simulink model "sampleModel1883"  (R2023a)
settings: Solver=VariableStepAuto  StartTime=0.0  StopTime=10.0  RelTol=1e-3
libraries: hdlsllib x1
settings Model: Creator=user1  LastModifiedBy=user1

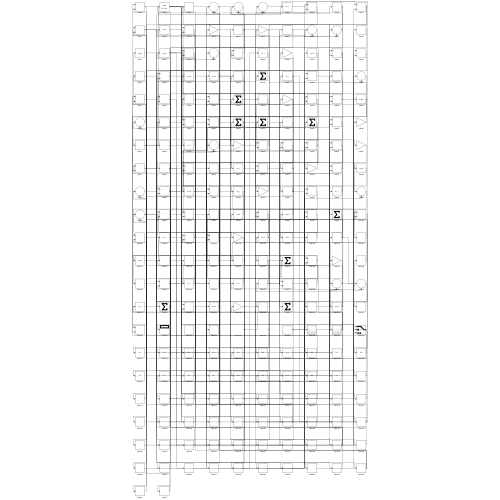
[thumbnail: Simulink's stored preview of the top-level diagram]
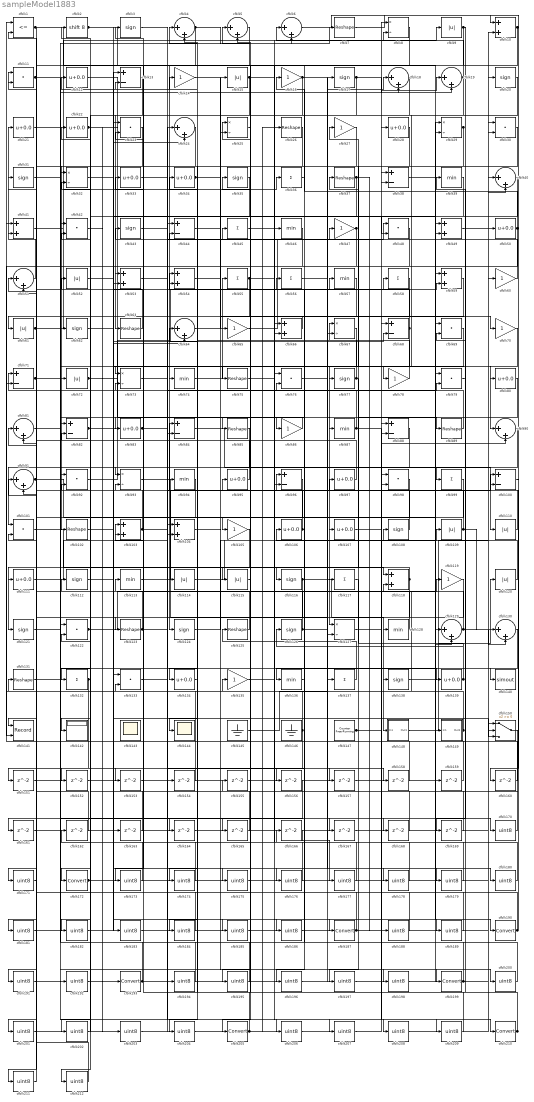
== system sampleModel1883 ==
  cfblk1 : RelationalOperator  Operator=<=  OutDataTypeStr=boolean  InputSameDT=off
  cfblk{10,41,49,53..54,59,66,103..104,118} (10 alike) : Sum
  cfblk{13,38,44,68,71,82,84,88,96,100} (10 alike) : Sum  Inputs=+-
  cfblk{11,23,30,42,48,69,76,79,92,98,101,122,133} (13 alike) : DotProduct  OutDataTypeStr=Inherit: Inherit via internal rule
  cfblk{7,26,37,63,75,85,89,102,123,125,131} (11 alike) : Reshape
  cfblk{14,16,27,47,60,65,70,78,86,105,119,135} (12 alike) : Gain
  cfblk{12,21..22,28,33..34,50,80,83,95,97,106..107,111,134,139} (16 alike) : Bias  Bias=0.0  SaturateOnIntegerOverflow=off
  cfblk{3,17,20,31,35,43,62,77,108,112,116,121,124,126,138} (15 alike) : Signum
  cfblk{9,15,52,61,72,109..110,114..115,120} (10 alike) : Abs  SaturateOnIntegerOverflow=off
  cfblk{39,46,57,74,87,94,113,128,136} (9 alike) : MinMax
  cfblk{36,45,55..56,58,99,117,132,137} (9 alike) : Sum  Inputs=+
  cfblk{8,25,29,32,67,73,93,127} (8 alike) : Product  Inputs=*/  RndMeth=Zero  SaturateOnIntegerOverflow=on
  cfblk{4..6,18..19,24,40,51,64,81,90..91,129..130} (14 alike) : Sum  Inputs=|++
  cfblk140 : ToWorkspace  VariableName=simout  SaveFormat=Timeseries  SampleTime=-1
  cfblk141 : Record  FileSettingsInternal="{\"entries\":[{\"content\":{\"excelSettings\":{\"content\":{},\"type\":\"Streamout.ExcelSettings\"}},\"type\":\"Streamout.FileSettingStorage\",\"uuid\":\"\"}],\"packageUris\":[\"http:\\/\\/schema.mathworks.com\\/mf0\\/streamout_blocks\\/R2020a\"],\"version\":\"1.0\"}"  Layout=[1 1]  SignalsInternal="{\"entries\":[{\"content\":{\"signals\":[{\"content\":{\"blockPath\":[],\"dimensions\":[1],\"domain\":\"\",\"lineColor\":\"#a2142f\",\"plots\":[1],\"port\":1,\"signalID\":4777,\"signalName\":\"XY Graph:1\"},\"type\":\"RecordBlkView.Signal\",\"uuid\":\"\"},{\"content\":{\"blockPath\":[],\"dimensions\":[1],\"domain\":\"\",\"lineColor\":\"#139fff\",\"plots\":[1],\"port\":2,\"signalID\":4780,\"signalName\":\"XY Graph:2\"},\"type\":\"RecordBlkView.Signal\",\"uuid\":\"\"}]},\"type\":\"RecordBlkView.InputSignals\",\"uuid\":\"\"}],\"packageUris\":[\"http:\\/\\/schema.mathworks.com\\/mf0\\/streamout_blocks\\/R2020a\"],\"version\":\"1.0\"}"  VisualizationBindings="{\"xyplotplugin\":{\"info\":[{\"series\":[{\"bindingParametersList\":[{\"parameter\":\"X-Axis\",\"signalID\":4777,\"signalName\":\"XY Graph:1\"},{\"parameter\":\"Y-Axis\",\"signalID\":4780,\"signalName\":\"XY Graph:2\"}],\"seriesID\":27607}],\"subplotID\":1}]}}"  CompatibilityTag=XY  st=-1
  cfblk142 : Display
  cfblk143 : Scope
      settings: Floating=on
  cfblk144 : Scope
  cfblk145 : Ground
  cfblk146 : Ground
  cfblk147 : hdlsllib/Sources/Counter Free-Running  NumBits=16  tsamp=-1
  cfblk148 : Subsystem
      settings: LibrarySourceBlock=|
      | hdlsllib/Ports &
      | Subsystems/Subsystem
  cfblk149 : Subsystem
      settings: LibrarySourceBlock=|
      | hdlsllib/Ports &
      | Subsystems/Subsystem
  cfblk150 : Switch  SaturateOnIntegerOverflow=off  InputSameDT=off
  cfblk{151..169} (19 alike) : Delay  SampleTime=1
  cfblk{170..171,173..186,188..189,191..192,194..198,200..204,206..209,211..212} (36 alike) : DataTypeConversion  OutDataTypeStr=uint8  SaturateOnIntegerOverflow=off  RndMeth=Floor
  cfblk{172,187,190,193,199,205,210} (7 alike) : DataTypeConversion  SaturateOnIntegerOverflow=off  RndMeth=Floor
  cfblk2 : ArithShift  BitShiftNumber=8
  wires:
  cfblk59/1 -> cfblk124/1
  cfblk67/1 -> cfblk127/1
  cfblk12/1 -> cfblk87/1
  cfblk147/1 -> cfblk90/2, cfblk179/1
  cfblk114/1 -> cfblk108/1
  cfblk70/1 -> cfblk90/1
  cfblk41/1 -> cfblk9/1
  cfblk18/1 -> cfblk63/1
  cfblk85/1 -> cfblk101/1
  cfblk11/1 -> cfblk19/2, cfblk206/1
  cfblk108/1 -> cfblk84/1
  cfblk109/1 -> cfblk71/1, cfblk130/1, cfblk73/2
  cfblk104/1 -> cfblk199/1
  cfblk105/1 -> cfblk121/1
  cfblk122/1 -> cfblk28/1, cfblk24/2
  cfblk89/1 -> cfblk51/1
  cfblk8/1 -> cfblk74/1
  cfblk146/1 -> cfblk101/2, cfblk212/1
  cfblk63/1 -> cfblk11/1
  cfblk74/1 -> cfblk55/1
  cfblk65/1 -> cfblk47/1
  cfblk101/1 -> cfblk118/1
  cfblk137/1 -> cfblk125/1
  cfblk79/1 -> cfblk39/1
  cfblk120/1 -> cfblk56/1
  cfblk26/1 -> cfblk102/1
  cfblk125/1 -> cfblk103/1
  cfblk87/1 -> cfblk27/1, cfblk64/1, cfblk200/1
  cfblk61/1 -> cfblk36/1, cfblk139/1
  cfblk129/1 -> cfblk25/1, cfblk130/2
  cfblk124/1 -> cfblk109/1
  cfblk149/1(Out1) -> cfblk14/1, cfblk112/1, cfblk118/2
  cfblk34/1 -> cfblk49/2, cfblk158/1
  cfblk37/1 -> cfblk53/1, cfblk188/1
  cfblk7/1 -> cfblk140/1
  cfblk73/1 -> cfblk105/1
  cfblk49/1 -> cfblk50/1
  cfblk15/1 -> cfblk73/1, cfblk189/1
  cfblk118/1 -> cfblk111/1, cfblk191/1
  cfblk111/1 -> cfblk24/1
  cfblk99/1 -> cfblk141/1
  cfblk47/1 -> cfblk71/2, cfblk195/1
  cfblk22/1 -> cfblk65/1, cfblk150/2, cfblk163/1
  cfblk66/1 -> cfblk61/1
  cfblk128/1 -> cfblk95/1
  cfblk24/1 -> cfblk132/1
  cfblk148/1(Out1) -> cfblk60/1
  cfblk38/1 -> cfblk190/1
  cfblk55/1 -> cfblk123/1, cfblk89/1
  cfblk126/1 -> cfblk119/1, cfblk52/1, cfblk18/1
  cfblk69/1 -> cfblk144/1
  cfblk86/1 -> cfblk82/1
  cfblk62/1 -> cfblk80/1
  cfblk98/1 -> cfblk205/1
  cfblk6/1 -> cfblk10/1
  cfblk92/1 -> cfblk58/1
  cfblk56/1 -> cfblk127/2
  cfblk115/1 -> cfblk45/1
  cfblk2/1 -> cfblk149/1(In1), cfblk48/2, cfblk75/1, cfblk150/3, cfblk64/2
  cfblk80/1 -> cfblk107/1
  cfblk119/1 -> cfblk148/1(In1)
  cfblk19/1 -> cfblk78/1, cfblk6/1
  cfblk121/1 -> cfblk62/1
  cfblk84/1 -> cfblk110/1
  cfblk54/1 -> cfblk70/1
  cfblk116/1 -> cfblk128/1, cfblk204/1
  cfblk93/1 -> cfblk137/1
  cfblk64/1 -> cfblk15/1
  cfblk78/1 -> cfblk37/1
  cfblk145/1 -> cfblk17/1
  cfblk91/1 -> cfblk129/1, cfblk198/1
  cfblk134/1 -> cfblk94/1
  cfblk113/1 -> cfblk8/1
  cfblk58/1 -> cfblk134/1
  cfblk139/1 -> cfblk67/1, cfblk126/1
  cfblk82/1 -> cfblk57/1, cfblk54/1
  cfblk102/1 -> cfblk68/2
  cfblk28/1 -> cfblk77/1
  cfblk123/1 -> cfblk59/2, cfblk31/1, cfblk100/1
  cfblk107/1 -> cfblk19/1
  cfblk25/1 -> cfblk5/2
  cfblk4/1 -> cfblk91/2, cfblk6/2
  cfblk77/1 -> cfblk12/1, cfblk117/1
  cfblk16/1 -> cfblk99/1, cfblk182/1
  cfblk138/1 -> cfblk120/1
  cfblk51/1 -> cfblk21/1
  cfblk33/1 -> cfblk115/1
  cfblk42/1 -> cfblk193/1
  cfblk81/1 -> cfblk210/1
  cfblk20/1 -> cfblk83/1
  cfblk44/1 -> cfblk187/1
  cfblk21/1 -> cfblk92/1
  cfblk95/1 -> cfblk11/2
  cfblk106/1 -> cfblk96/1, cfblk156/1
  cfblk50/1 -> cfblk16/1, cfblk141/2, cfblk53/2
  cfblk110/1 -> cfblk97/1
  cfblk72/1 -> cfblk114/1, cfblk2/1, cfblk203/1
  cfblk103/1 -> cfblk41/2, cfblk185/1
  cfblk39/1 -> cfblk96/2
  cfblk68/1 -> cfblk72/1, cfblk54/2
  cfblk97/1 -> cfblk35/1
  cfblk60/1 -> cfblk3/1
  cfblk83/1 -> cfblk48/1, cfblk79/2
  cfblk75/1 -> cfblk8/2
  cfblk57/1 -> cfblk85/1
  cfblk10/1 -> cfblk86/1, cfblk165/1
  cfblk36/1 -> cfblk116/1
  cfblk132/1 -> cfblk22/1, cfblk161/1
  cfblk1/1 -> cfblk46/1, cfblk211/1
  cfblk17/1 -> cfblk25/2, cfblk18/2
  cfblk13/1 -> cfblk172/1
  cfblk130/1 -> cfblk136/1
  cfblk29/1 -> cfblk142/1, cfblk66/2
  cfblk71/1 -> cfblk138/1, cfblk7/1
  cfblk9/1 -> cfblk29/2, cfblk169/1
  cfblk136/1 -> cfblk106/1
  cfblk5/1 -> cfblk93/1
  cfblk94/1 -> cfblk151/1
  cfblk151/1 -> cfblk29/1
  cfblk35/1 -> cfblk152/1
  cfblk152/1 -> cfblk84/2
  cfblk96/1 -> cfblk153/1
  cfblk133/1 -> cfblk154/1
  cfblk154/1 -> cfblk1/1
  cfblk150/1 -> cfblk155/1
  cfblk155/1 -> cfblk5/1
  cfblk53/1 -> cfblk157/1
  cfblk157/1 -> cfblk129/2
  cfblk158/1 -> cfblk91/1
  cfblk159/1 -> cfblk122/2
  cfblk100/1 -> cfblk160/1
  cfblk160/1 -> cfblk41/1
  cfblk161/1 -> cfblk10/2
  cfblk162/1 -> cfblk1/2
  cfblk163/1 -> cfblk82/2
  cfblk90/1 -> cfblk164/1
  cfblk164/1 -> cfblk59/1
  cfblk165/1 -> cfblk103/2
  cfblk43/1 -> cfblk167/1
  cfblk167/1 -> cfblk68/1
  cfblk45/1 -> cfblk168/1
  cfblk168/1 -> cfblk66/1
  cfblk169/1 -> cfblk93/2
  cfblk131/1 -> cfblk170/1
  cfblk170/1 -> cfblk133/1
  cfblk27/1 -> cfblk171/1
  cfblk171/1 -> cfblk131/1
  cfblk172/1 -> cfblk79/1, cfblk186/1
  cfblk48/1 -> cfblk173/1
  cfblk173/1 -> cfblk13/1
  cfblk46/1 -> cfblk174/1
  cfblk174/1 -> cfblk13/2
  cfblk32/1 -> cfblk175/1
  cfblk175/1 -> cfblk20/1
  cfblk14/1 -> cfblk176/1
  cfblk176/1 -> cfblk32/1
  cfblk166/1 -> cfblk177/1
  cfblk177/1 -> cfblk32/2
  cfblk76/1 -> cfblk178/1
  cfblk178/1 -> cfblk43/1
  cfblk179/1 -> cfblk76/1
  cfblk112/1 -> cfblk180/1
  cfblk180/1 -> cfblk76/2
  cfblk23/1 -> cfblk181/1
  cfblk181/1 -> cfblk159/1
  cfblk182/1 -> cfblk23/1
  cfblk52/1 -> cfblk183/1
  cfblk183/1 -> cfblk23/2
  cfblk30/1 -> cfblk184/1
  cfblk184/1 -> cfblk122/1
  cfblk185/1 -> cfblk30/1
  cfblk186/1 -> cfblk30/2
  cfblk187/1 -> cfblk133/2, cfblk51/2
  cfblk188/1 -> cfblk44/1
  cfblk189/1 -> cfblk44/2
  cfblk190/1 -> cfblk100/2, cfblk34/1
  cfblk191/1 -> cfblk38/1
  cfblk31/1 -> cfblk192/1
  cfblk192/1 -> cfblk38/2
  cfblk193/1 -> cfblk162/1, cfblk67/2
  cfblk3/1 -> cfblk194/1
  cfblk194/1 -> cfblk42/1
  cfblk195/1 -> cfblk42/2
  cfblk40/1 -> cfblk196/1
  cfblk196/1 -> cfblk69/1
  cfblk117/1 -> cfblk197/1
  cfblk197/1 -> cfblk40/1
  cfblk198/1 -> cfblk40/2
  cfblk199/1 -> cfblk166/1, cfblk49/1, cfblk113/1
  cfblk200/1 -> cfblk104/1
  cfblk156/1 -> cfblk201/1
  cfblk201/1 -> cfblk104/2
  cfblk88/1 -> cfblk202/1
  cfblk202/1 -> cfblk92/2
  cfblk203/1 -> cfblk88/1
  cfblk204/1 -> cfblk88/2
  cfblk205/1 -> cfblk33/1, cfblk26/1
  cfblk206/1 -> cfblk98/1
  cfblk153/1 -> cfblk207/1
  cfblk207/1 -> cfblk98/2
  cfblk135/1 -> cfblk208/1
  cfblk208/1 -> cfblk150/1
  cfblk127/1 -> cfblk209/1
  cfblk209/1 -> cfblk135/1
  cfblk210/1 -> cfblk4/2, cfblk4/1, cfblk69/2
  cfblk211/1 -> cfblk81/1
  cfblk212/1 -> cfblk81/2

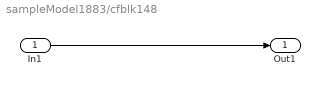
== system sampleModel1883/cfblk148 ==
  In1 : Inport
  Out1 : Outport
  wires:
  In1/1 -> Out1/1

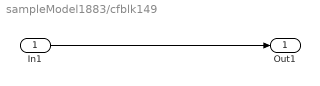
== system sampleModel1883/cfblk149 ==
  In1 : Inport
  Out1 : Outport
  wires:
  In1/1 -> Out1/1
